simulink model "main"  (R2024a)
settings: Solver=VariableStepAuto  StartTime=0.0  StopTime=100  RelTol=1e-3
settings Model: Creator=filip  LastModifiedBy=raden

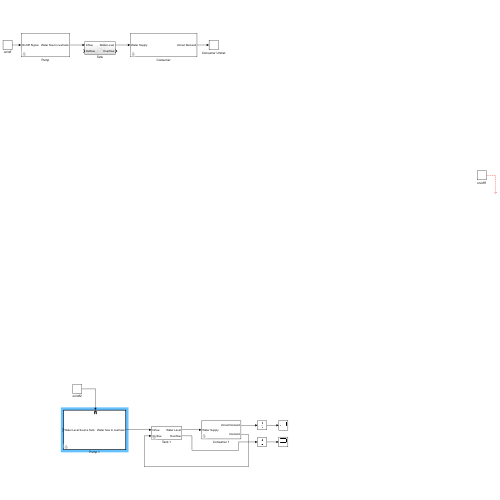
[thumbnail: Simulink's stored preview of the top-level diagram]
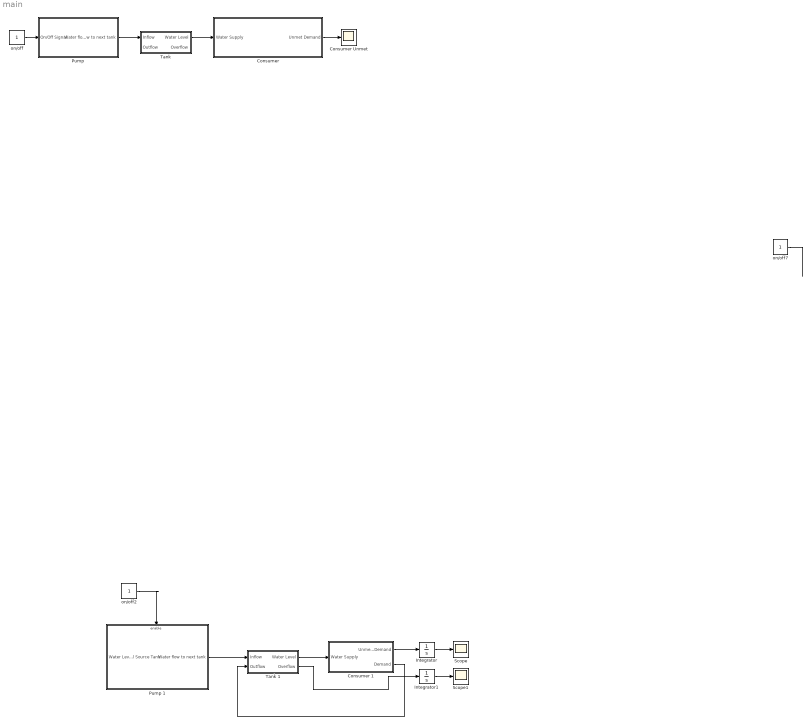
== system main ==
  Consumer : Subsystem  mask{a_i=5, f_i=1, d_i=20}
  Consumer 1 : Subsystem  mask{a_i=3.0, f_i=0.4, d_i=2.0}
      mask prompts: f_i "frequenz"; d_i "delay"
  Consumer Unmet : Scope
  Integrator : Integrator
  Integrator1 : Integrator
  Pump : Subsystem  mask{p_i=200}
  Pump 1 : Subsystem  TreatAsAtomicUnit=on  mask{p_i=15}
      mask prompts: p_i "volume per Time (p_i)"
  Scope : Scope
  Scope1 : Scope
  Tank : Subsystem
  Tank 1 : Subsystem  mask{c_i=100, c_i_init=50}
      mask prompts: c_i "capacity (c_i)"; c_i_init "Init capacity (c_i_init)"
  on/off : Constant
  on/off2 : Constant
  on/off7 : Constant
  wires:
  Pump/1(Water flow to next tank) -> Tank/1(Inflow)
  on/off/1 -> Pump/1(On/Off Signal)
  Tank/1(Water Level) -> Consumer/1(Water Supply)
  Consumer/1(Unmet Demand) -> Consumer Unmet/1
  Pump 1/1(Water flow to next tank) -> Tank 1/1(Inflow)
  Tank 1/1(Water Level) -> Consumer 1/1(Water Supply)
  on/off7/1 -> ?
  on/off2/1 -> Pump 1/Enable
  Consumer 1/2(Demand) -> Tank 1/2(Outflow)
  Consumer 1/1(Unmet Demand) -> Integrator/1
  Tank 1/2(Overflow) -> Integrator1/1
  Integrator/1 -> Scope/1
  Integrator1/1 -> Scope1/1

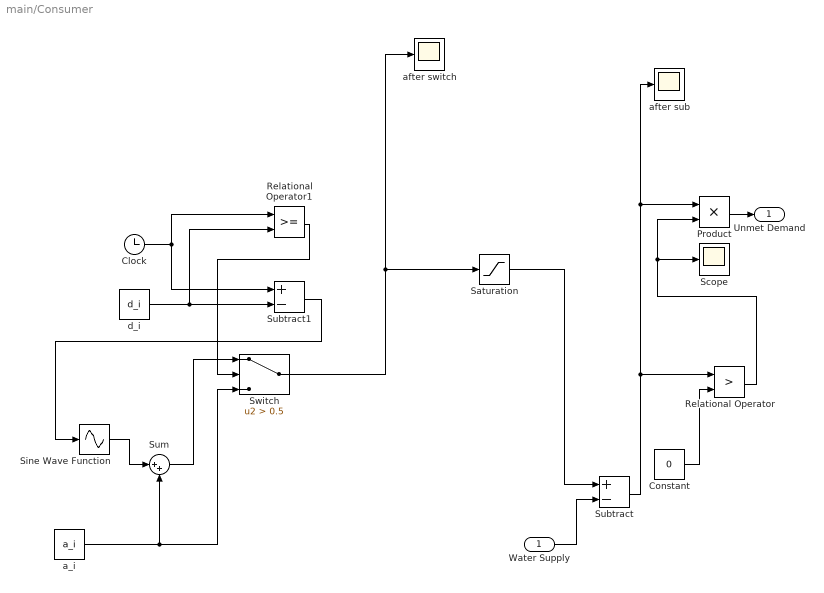
== system main/Consumer ==
  Water Supply : Inport
  Clock : Clock
  Constant : Constant  Value=0
  Product : Product
  Relational Operator : RelationalOperator  Operator=>  OutDataTypeStr=boolean  RndMeth=Simplest  InputSameDT=off
  Relational Operator1 : RelationalOperator  OutDataTypeStr=boolean  RndMeth=Simplest  InputSameDT=off
  Saturation : Saturate  UpperLimit=inf  LowerLimit=0
  Scope : Scope
  Sine Wave Function : Sin  TimeSource=Use external signal  Amplitude=a_i  Frequency=f_i  SampleTime=0
  Subtract : Sum  Inputs=+-
  Subtract1 : Sum  Inputs=+-
  Sum : Sum  Inputs=|++
  Switch : Switch  Criteria=u2 > Threshold  Threshold=0.5  SaturateOnIntegerOverflow=off  InputSameDT=off
  a_i : Constant  Value=a_i
  after sub : Scope
  after switch : Scope
  d_i : Constant  Value=d_i
  Unmet Demand : Outport
  wires:
  a_i/1 -> Sum/2, Switch/3
  Water Supply/1 -> Subtract/2
  Subtract/1 -> Relational Operator/1, after sub/1, Product/1
  Relational Operator/1 -> Scope/1, Product/2
  Product/1 -> Unmet Demand/1
  Switch/1 -> after switch/1, Saturation/1
  Saturation/1 -> Subtract/1
  Constant/1 -> Relational Operator/2
  Clock/1 -> Relational Operator1/1, Subtract1/1
  d_i/1 -> Relational Operator1/2, Subtract1/2
  Subtract1/1 -> Sine Wave Function/1
  Relational Operator1/1 -> Switch/2
  Sum/1 -> Switch/1
  Sine Wave Function/1 -> Sum/1

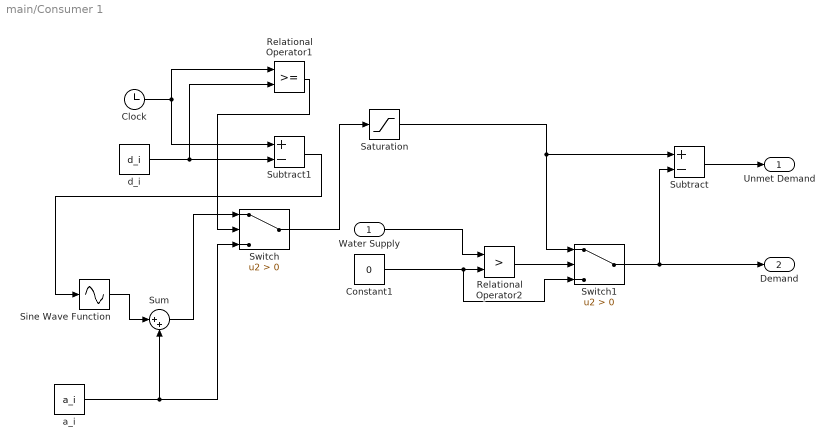
== system main/Consumer 1 ==
  Water Supply : Inport
  Clock : Clock
  Constant1 : Constant  Value=0
  Relational Operator1 : RelationalOperator  OutDataTypeStr=boolean  RndMeth=Simplest  InputSameDT=off
  Relational Operator2 : RelationalOperator  Operator=>  OutDataTypeStr=boolean  RndMeth=Simplest  InputSameDT=off
  Saturation : Saturate  UpperLimit=inf  LowerLimit=0
  Sine Wave Function : Sin  TimeSource=Use external signal  Amplitude=a_i  Frequency=f_i  SampleTime=0
  Subtract : Sum  Inputs=+-
  Subtract1 : Sum  Inputs=+-
  Sum : Sum  Inputs=|++
  Switch : Switch  Criteria=u2 > Threshold  SaturateOnIntegerOverflow=off  InputSameDT=off
  Switch1 : Switch  Criteria=u2 > Threshold  SaturateOnIntegerOverflow=off  InputSameDT=off
  a_i : Constant  Value=a_i
  d_i : Constant  Value=d_i
  Unmet Demand : Outport
  Demand : Outport  Port=2
  wires:
  a_i/1 -> Sum/2, Switch/3
  Switch/1 -> Saturation/1
  Saturation/1 -> Subtract/1, Switch1/1
  Clock/1 -> Relational Operator1/1, Subtract1/1
  d_i/1 -> Relational Operator1/2, Subtract1/2
  Subtract1/1 -> Sine Wave Function/1
  Relational Operator1/1 -> Switch/2
  Sum/1 -> Switch/1
  Sine Wave Function/1 -> Sum/1
  Water Supply/1 -> Relational Operator2/1
  Constant1/1 -> Relational Operator2/2, Switch1/3
  Relational Operator2/1 -> Switch1/2
  Switch1/1 -> Subtract/2, Demand/1
  Subtract/1 -> Unmet Demand/1

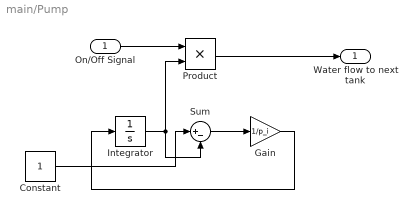
== system main/Pump ==
  On/Off Signal : Inport
  Constant : Constant
  Gain : Gain  Gain=1/p_i
  Integrator : Integrator
  Product : Product
  Sum : Sum  Inputs=|+-
  Water flow to next tank : Outport
  wires:
  Integrator/1 -> Product/2, Sum/2
  On/Off Signal/1 -> Product/1
  Product/1 -> Water flow to next tank/1
  Constant/1 -> Sum/1
  Sum/1 -> Gain/1
  Gain/1 -> Integrator/1

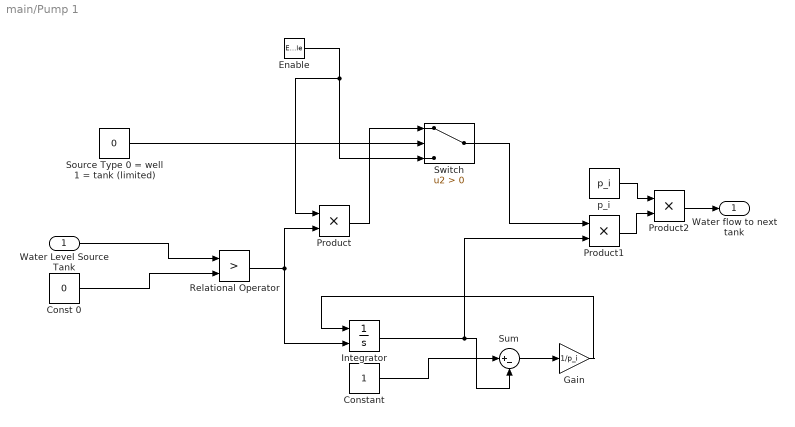
== system main/Pump 1 ==
  Water Level Source Tank : Inport
  Enable : EnablePort  ShowOutputPort=on
  Const 0 : Constant  Value=0
  Constant : Constant
  Gain : Gain  Gain=1/p_i
  Integrator : Integrator  ExternalReset=falling
  Product : Product
  Product1 : Product
  Product2 : Product
  Relational Operator : RelationalOperator  Operator=>  OutDataTypeStr=boolean  RndMeth=Simplest  InputSameDT=off
  Source Type 0 = well 1 = tank (limited) : Constant  Value=0
  Sum : Sum  Inputs=|+-
  Switch : Switch  Criteria=u2 > Threshold  SaturateOnIntegerOverflow=off  InputSameDT=off
  p_i : Constant  Value=p_i
  Water flow to next tank : Outport
  wires:
  Sum/1 -> Gain/1
  Integrator/1 -> Sum/2, Product1/2
  Constant/1 -> Sum/1
  Gain/1 -> Integrator/1
  Enable/1 -> Switch/3, Product/1
  Source Type 0 = well 1 = tank (limited)/1 -> Switch/2
  Water Level Source Tank/1 -> Relational Operator/1
  Const 0/1 -> Relational Operator/2
  Relational Operator/1 -> Integrator/2, Product/2
  Switch/1 -> Product1/1
  Product/1 -> Switch/1
  Product1/1 -> Product2/2
  p_i/1 -> Product2/1
  Product2/1 -> Water flow to next tank/1

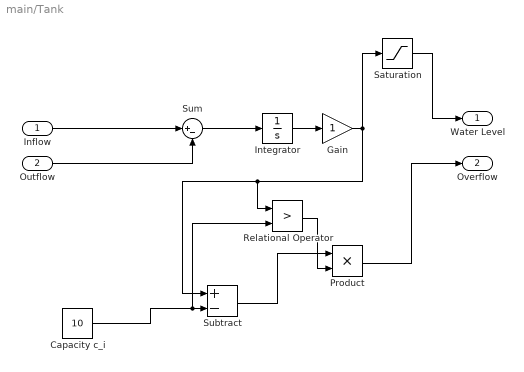
== system main/Tank ==
  Inflow : Inport
  Outflow : Inport  Port=2
  Capacity c_i : Constant  Value=10
  Gain : Gain
  Integrator : Integrator
  Product : Product
  Relational Operator : RelationalOperator  Operator=>  OutDataTypeStr=boolean  RndMeth=Simplest  InputSameDT=off
  Saturation : Saturate  UpperLimit=10  LowerLimit=0
  Subtract : Sum  Inputs=+-
  Sum : Sum  Inputs=|+-
  Water Level : Outport
  Overflow : Outport  Port=2
  wires:
  Inflow/1 -> Sum/1
  Outflow/1 -> Sum/2
  Sum/1 -> Integrator/1
  Integrator/1 -> Gain/1
  Gain/1 -> Relational Operator/1, Subtract/1, Saturation/1
  Capacity c_i/1 -> Relational Operator/2, Subtract/2
  Saturation/1 -> Water Level/1
  Product/1 -> Overflow/1
  Subtract/1 -> Product/1
  Relational Operator/1 -> Product/2

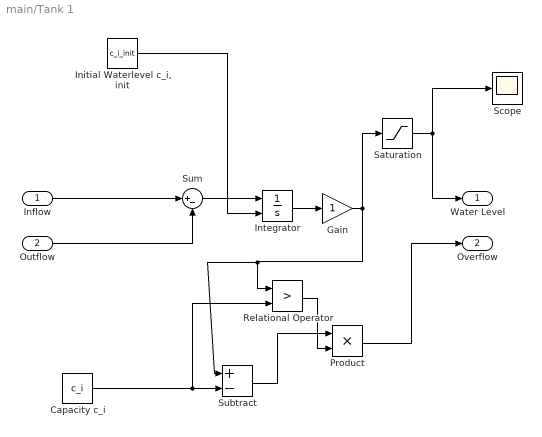
== system main/Tank 1 ==
  Inflow : Inport
  Outflow : Inport  Port=2
  Capacity c_i : Constant  Value=c_i
  Gain : Gain
  "Initial Waterlevel c_i, init" : Constant  Value=c_i_init
  Integrator : Integrator  InitialConditionSource=external
  Product : Product
  Relational Operator : RelationalOperator  Operator=>  OutDataTypeStr=boolean  RndMeth=Simplest  InputSameDT=off
  Saturation : Saturate  UpperLimit=100  LowerLimit=0
  Scope : Scope
  Subtract : Sum  Inputs=+-
  Sum : Sum  Inputs=|+-
  Water Level : Outport
  Overflow : Outport  Port=2
  wires:
  Inflow/1 -> Sum/1
  Outflow/1 -> Sum/2
  Sum/1 -> Integrator/1
  Integrator/1 -> Gain/1
  Gain/1 -> Relational Operator/1, Subtract/1, Saturation/1
  Capacity c_i/1 -> Relational Operator/2, Subtract/2
  Saturation/1 -> Scope/1, Water Level/1
  Product/1 -> Overflow/1
  Subtract/1 -> Product/1
  Relational Operator/1 -> Product/2
  "Initial Waterlevel c_i, init"/1 -> Integrator/2
